simulink model "second"  (R2023b)
settings: Solver=VariableStepAuto  StartTime=0.0  StopTime=10  RelTol=1e-3
values from neighbouring files (symbols this model uses):
  L = -P*(eye(size(Q)) - gamma^(-2)*Q*P)^-1*(C_1+gamma^(-2)*D_1*B_1'*Q)'*(D_1*D_1')^-1    [Hinf_controller_observer.m]
undefined symbols (not defined in the file or in its folder): A, B_1, B_2, C_1, C_2, C_21, D_1, D_2, D_21, K_1, K_2, x_0
settings Model: Creator=evdokiiagalkina  LastModifiedBy=evdokiiagalkina

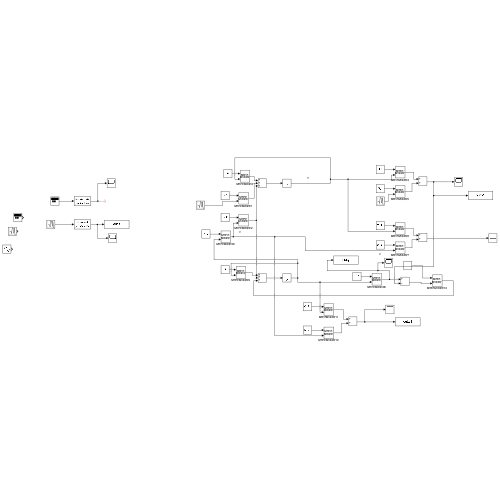
[thumbnail: Simulink's stored preview of the top-level diagram]
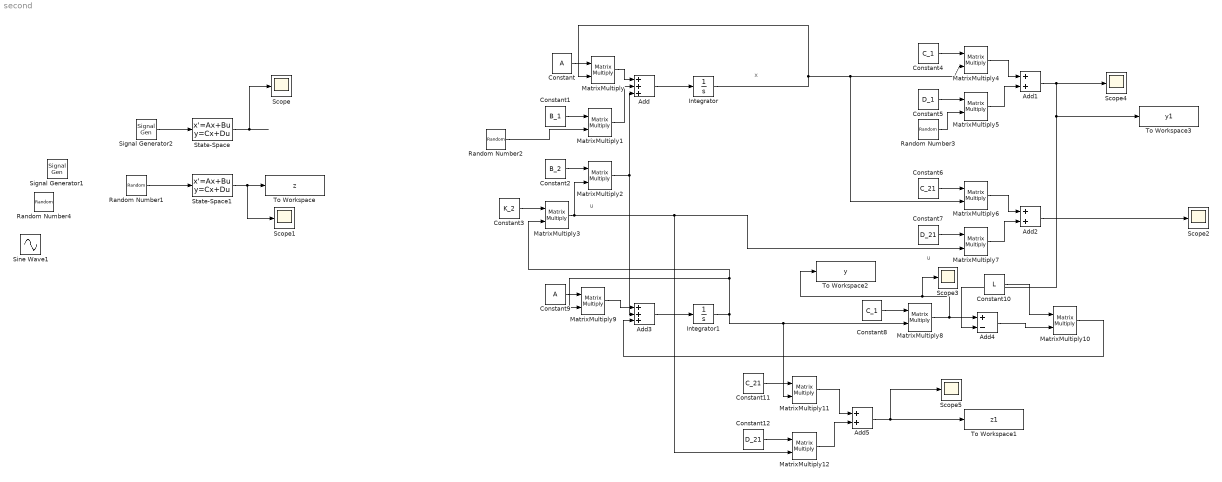
== system second ==
  note: u
  note: x
  note: u
  Add : Sum  Inputs=+++
  Add1 : Sum
  Add2 : Sum
  Add3 : Sum  Inputs=+++
  Add4 : Sum  Inputs=+-
  Add5 : Sum
  Constant : Constant  Value=A
  Constant1 : Constant  Value=B_1
  Constant10 : Constant  Value=L  VectorParams1D=off
  Constant11 : Constant  Value=C_21  VectorParams1D=off
  Constant12 : Constant  Value=D_21  VectorParams1D=off
  Constant2 : Constant  Value=B_2  VectorParams1D=off
  Constant3 : Constant  Value=K_2  VectorParams1D=off
  Constant4 : Constant  Value=C_1  VectorParams1D=off
  Constant5 : Constant  Value=D_1  VectorParams1D=off
  Constant6 : Constant  Value=C_21  VectorParams1D=off
  Constant7 : Constant  Value=D_21  VectorParams1D=off
  Constant8 : Constant  Value=C_1  VectorParams1D=off
  Constant9 : Constant  Value=A  VectorParams1D=off
  Integrator : Integrator  InitialCondition=x_0
  Integrator1 : Integrator  InitialCondition=[0; 0]
  MatrixMultiply{,1..12} (13 alike) : Product  Multiplication=Matrix(*)
  Random Number{1..4} (4 alike) : RandomNumber  SampleTime=0.001
  Scope{,1..5} (6 alike) : Scope
  Signal Generator1 : SignalGenerator  WaveForm=square  Amplitude=0.1  Frequency=5  Units=rad/sec
  Signal Generator2 : SignalGenerator  WaveForm=square  Amplitude=0.1  Frequency=5  Units=rad/sec
  Sine Wave1 : Sin  SampleTime=0
  State-Space : StateSpace  A=[A, B_2*K_1;-L*C_1,A+B_2*K_1+L*C_1]  B=[B_1; -L*D_1]  C=[C_2, D_2*K_1]  D=zeros(size(C_2, 1), size(B_1, 2))  InitialCondition=[x_0, 0*x_0]
  State-Space1 : StateSpace  A=[A, B_2*K_2;-L*C_1,A+B_2*K_2+L*C_1]  B=[B_1; -L*D_1]  C=[C_21 D_21*K_2]  D=zeros(size(C_21, 1), size(B_1, 2))  InitialCondition=[x_0, 0*x_0]
  To Workspace : ToWorkspace  VariableName=z  SaveFormat=Timeseries  SampleTime=-1
  To Workspace1 : ToWorkspace  VariableName=z1  SaveFormat=Timeseries  SampleTime=-1
  To Workspace2 : ToWorkspace  VariableName=y  SaveFormat=Timeseries  SampleTime=-1
  To Workspace3 : ToWorkspace  VariableName=y1  SaveFormat=Timeseries  SampleTime=-1
  wires:
  Signal Generator2/1 -> State-Space/1
  Random Number1/1 -> State-Space1/1
  State-Space/1 -> Scope/1
  State-Space1/1 -> To Workspace/1, Scope1/1
  Add/1 -> Integrator/1
  Constant/1 -> MatrixMultiply/1
  MatrixMultiply/1 -> Add/1
  Constant1/1 -> MatrixMultiply1/1
  Constant2/1 -> MatrixMultiply2/1
  MatrixMultiply1/1 -> Add/2
  MatrixMultiply2/1 -> Add3/2, Add/3
  Integrator/1 -> MatrixMultiply/2, MatrixMultiply4/2, MatrixMultiply6/2
  Random Number2/1 -> MatrixMultiply1/2
  Constant3/1 -> MatrixMultiply3/1
  MatrixMultiply3/1 -> MatrixMultiply12/2, MatrixMultiply7/2, MatrixMultiply2/2
  Constant4/1 -> MatrixMultiply4/1
  Constant5/1 -> MatrixMultiply5/1
  Random Number3/1 -> MatrixMultiply5/2
  MatrixMultiply4/1 -> Add1/1
  MatrixMultiply5/1 -> Add1/2
  Integrator1/1 -> MatrixMultiply9/2, MatrixMultiply3/2, MatrixMultiply11/2, MatrixMultiply8/2
  MatrixMultiply6/1 -> Add2/1
  MatrixMultiply7/1 -> Add2/2
  Constant6/1 -> MatrixMultiply6/1
  Constant7/1 -> MatrixMultiply7/1
  Constant8/1 -> MatrixMultiply8/1
  Add3/1 -> Integrator1/1
  Constant9/1 -> MatrixMultiply9/1
  MatrixMultiply9/1 -> Add3/1
  MatrixMultiply8/1 -> To Workspace2/1, Scope3/1, Add4/1
  Add1/1 -> Scope4/1, To Workspace3/1, Add4/2
  Constant10/1 -> MatrixMultiply10/1
  Add4/1 -> MatrixMultiply10/2
  MatrixMultiply10/1 -> Add3/3
  Add2/1 -> Scope2/1
  Constant11/1 -> MatrixMultiply11/1
  Constant12/1 -> MatrixMultiply12/1
  MatrixMultiply11/1 -> Add5/1
  MatrixMultiply12/1 -> Add5/2
  Add5/1 -> Scope5/1, To Workspace1/1
